simulink model "sm_car_Unreal_Engine_test_transforms_R19b"  (R2021b)
settings: Solver=VariableStepAuto  StartTime=0.0  StopTime=20  RelTol=1e-3  EnableMultiTasking=on
undefined symbols (not defined in the file or in its folder): Newton, Raphson, X, Y, Z
libraries: sm_lib x18, nesl_utility x9, sharedtransformsys x3, sim3dlib x1, sim3dautolib x1, Vehicle_Visualization x1
Description:
  | Copyright 2020-2021 The MathWorks, Inc.
settings Model: Creator=bmirtich  LastModifiedBy=smiller
settings SolverCC: AlgebraicLoopSolver=TrustRegion
settings DataIOCC: LimitDataPoints=on  MaxDataPoints=10000
settings OptimizationCC: LifeSpan=inf
settings DebuggingCC: ParameterPrecisionLossMsg=none  ParameterTunabilityLossMsg=none  AllowSymbolicDim=off  SFUnexpectedBacktrackingDiag=warning  SFNoUnconditionalDefaultTransitionDiag=warning  SFExecutionAtInitializationDiag=none  SFMachineParentedDataDiag=warning  ArithmeticOperatorsInVariantConditions=warning
settings SFSimCC: SimUseLocalCustomCode=off  CustomCodeUndefinedFunction=UseInterfaceOnly
settings RTWCC: RTWUseLocalCustomCode=off
settings CodeAppCC: StateflowObjectComments=on
settings GRTTargetCC: TargetLangStandard=C89/C90 (ANSI)
settings ConfigComp: CovMetricSettings=dw  CovSaveCumulativeToWorkspaceVar=on  CovSaveSingleToWorkspaceVar=on  CovExternalEMLEnable=off  CovSFcnEnable=off
settings SimscapeCC: SimscapeLogType=all  SimscapeLogSimulationStatistics=on  SimscapeLogDataHistory=10000
settings DiagnosticsConfigSet: SimMechanicsConflictingReferenceFrames=none
settings ExplorerConfigSet: InternalSimMechanicsExplorerSettings="<ExplorerConfiguration><canonicalview>default</canonicalview><AnimationSetting><BasePlaybackSpeed>1.0</BasePlaybackSpeed><PlaybackSpeedFactor>2.0</PlaybackSpeedFactor></AnimationSetting><TilePanel><TileInfo><Tiles Columns=\"1\" Count=\"1\" Rows=\"1\"><Column Weight=\"1\"/><Row Weight=\"1\"/><Tile Height=\"1\" Width=\"1\" X=\"0\" Y=\"0\"/></Tiles></TileInfo><SceneInfo><SceneViewer><BGColor><R>1</R><G>1</G><B>1</B></BGColor><Camera><DoPerspective>on</DoPerspective><Position><X>-10</X><Y>0</Y><Z>1</Z></Position><Center><X>-9</X><Y>0</Y><Z>1</Z></Center><Up><X>0</X><Y>0</Y><Z>1</Z></Up><ViewLimDist>1</ViewLimDist><YLim>0.466307658154998583</YLim><XLim>0.637328144918969053</XLim></Camera></SceneViewer></SceneInfo></TilePanel><MechEditorPanel><Cameras><Camera><Id>Camera8</Id><Value><Name>Track Align Rear STL</Name><NativeCamera><PositionTrackingFeature>Vehicle_Geometry.Transform_Camera_Rear.F</PositionTrackingFeature><CenterTrackingFeature>Vehicle_Geometry.Transform_Camera_Rear.F</CenterTrackingFeature><UpVectorTrackingFeature>Vehicle_Geometry.Transform_Camera_Rear.F</UpVectorTrackingFeature><CenterTrackingOrigin>off</CenterTrackingOrigin><CenterTrackingDirection>+X</CenterTrackingDirection><UpVectorTrackingDirection>+Z</UpVectorTrackingDirection></NativeCamera></Value></Camera><Camera><Id>Camera9</Id><Value><Name>Track Rear Fixed View</Name><NativeCamera><PositionTrackingFeature>Ground_Plane.Transform_Camera_Fixed.F</PositionTrackingFeature><CenterTrackingFeature>Ground_Plane.Transform_Camera_Fixed.F</CenterTrackingFeature><UpVectorTrackingFeature>Ground_Plane.Transform_Camera_Fixed.F</UpVectorTrackingFeature><CenterTrackingOrigin>off</CenterTrackingOrigin><CenterTrackingDirection>+X</CenterTrackingDirection><UpVectorTrackingDirection>+Z</UpVectorTrackingDirection></NativeCamera></Value></Camera></Cameras><GfxPanelCameraMap><MapElement CameraMLId=\"Camera9\" GfxPanelIndex=\"0\"/></GfxPanelCameraMap><VideoCreator><PlaybackSpeedRatio>1.0</PlaybackSpeedRatio><FrameRate>30</FrameRate><VideoFormat>Motion JPEG AVI</VideoFormat><FrameSize>auto</FrameSize></VideoCreator></MechEditorPanel></ExplorerConfiguration>"

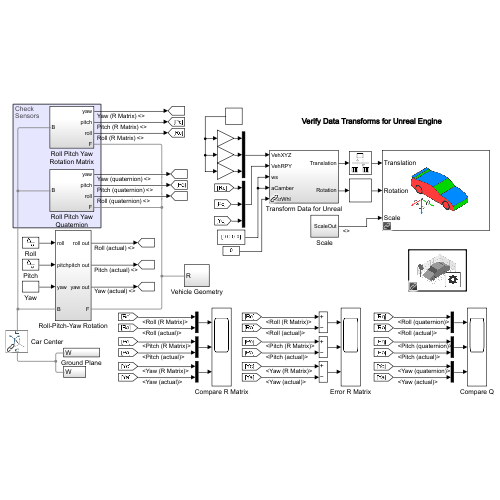
[thumbnail: Simulink's stored preview of the top-level diagram]
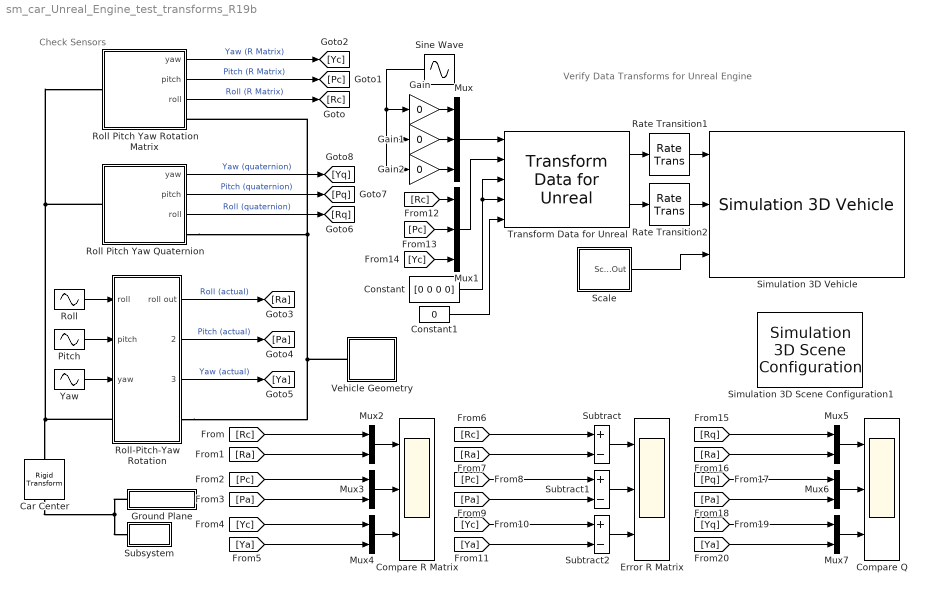
== system sm_car_Unreal_Engine_test_transforms_R19b ==
  note: Check
      | Sensors
  note: Verify Data Transforms for Unreal Engine
  Car Center : sm_lib/Frames and Transforms/Rigid Transform  TranslationMethod=Cartesian  TranslationStandardOffset=0  TranslationLengthUnit=m  TranslationStandardAxis=+Z  TranslationCartesianOffset=[0 0 .85]  TranslationROffset=0  TranslationROffsetUnits=m  TranslationZOffset=0  TranslationZOffsetUnits=m  TranslationThetaOffset=0  TranslationThetaOffsetUnits=deg  RotationMethod=None  RotationAngleUnits=deg  RotationStandardAxis=+Z  RotationAngle=0.0  RotationArbitraryAxis=[0 0 1]  FollAlignAxisA=+X  BaseAlignAxisA=+Y  FollAlignAxisB=+Y  BaseAlignAxisB=+Z  RotationSequenceAxes=FollowerAxes  RotationSequence=XYX  RotationSequenceAngles=[0 0 0]  RotationSequenceAnglesUnits=deg  RotationMatrix=[1 0 0; 0 1 0; 0 0 1]
      settings: SourceProductName=Multibody
  Compare Q : Scope  NumInputPorts=3
  Compare R Matrix : Scope  NumInputPorts=3
  Constant : Constant  Value=[0 0 0 0]
  Constant1 : Constant  Value=0
  Error R Matrix : Scope  NumInputPorts=3
  Gain : Gain  Gain=0
  Gain1 : Gain  Gain=0
  Gain2 : Gain  Gain=0
  Ground Plane : Subsystem
  Mux : Mux  Inputs=3
  Mux1 : Mux  Inputs=3
  Mux{2..7} (6 alike) : Mux  Inputs=2
  Pitch : Sin  Amplitude=80  Frequency=1.329  SampleTime=0
  Rate Transition1 : RateTransition  Deterministic=off  OutPortSampleTime=0.03
  Rate Transition2 : RateTransition  Deterministic=off  OutPortSampleTime=0.03
  Roll : Sin  Amplitude=150  Frequency=.991  SampleTime=0
  Roll Pitch Yaw Quaternion : Subsystem
  Roll Pitch Yaw Rotation Matrix : Subsystem
  Roll-Pitch-Yaw Rotation : Subsystem
  Scale : Subsystem
  Simulation 3D Scene Configuration1 : sim3dlib/Simulation 3D Scene Configuration  Priority=0  ProjectFormat_internal=Default Scenes  ProjectFormat=Default Scenes  SceneDesc=Double lane change  ProjectName=C:\Program Files\MATLAB\R2021b\toolbox\shared\sim3d_projects\automotive_project\UE4\WindowsNoEditor\VehicleSimulation.exe  ScenePath=/Game/Maps/HwStrght  vehTagList={'Scene Origin'}  vehTag=Scene Origin  OpVisEn=off  Ts=.03  EnableWindow=on  EnableWeather=off  SunAltitude=40.0  SunAzimuth=90  clouds=10  wind=1  fog=0  rain=0  sensorTag=MainCamera1  sensorId=1  sensorName=MainCamera1  mountLoc=Origin  offsetFlag=off  tmountOffset=[0, 0, 0]  rmountOffset=[0, 0, 0]  HorizontalResolution=1280  VerticalResolution=720  HorizontalFOV=60  mountPoint=[0 0 0]  mountOrientation=[0 0 0]  aMode=aMode  ID=1
      settings: SourceProductBaseCode=AE,DR,UV,VE
  Simulation 3D Vehicle : sim3dautolib/Simulation 3D Vehicle  Priority=-1  PassVehMesh=Muscle car  PassVehMesh_Internal=Muscle car  MeshPath=/MathWorksSimulation/Vehicles/Muscle/Meshes/SK_MuscleCar.SK_MuscleCar  VehColor=Red  VehColor_Internal=Red  ActorName=SimulinkVehicle1  VehLightsControl=off  HeadlightColor=[ 1, 1, 1 ]  HighBeamIntensity=100000  LowBeamIntensity=60000  HighBeamConeAngle=1.22  LowBeamConeAngle=1.22  LeftHeadlightOrientation=[ 0, 0 ]  RightHeadlightOrientation=[ 0, 0 ]  BrakelightIntensity=500  ReverselightIntensity=500  SignallightIntensity=500  SignallightPeriod=1  SignalPulseWidth=50  Translation=[0 0 1; 0 0 0; 0 0 0; 0 0 0; 0 0 0]  Rotation=[0 0 0; 0 0 0; 0 0 0; 0 0 0; 0 0 0]  Scale=ones( 5, 3 )  SampleTime=.03  ActorType=SimulinkVehicle  ID=1  aMode=2  ActorTag=SimulinkVehicle1
      settings: SourceProductBaseCode=AE,DR,UV,VE
  Sine Wave : Sin  SampleTime=0
  Subsystem : Subsystem
  Subtract : Sum  Inputs=+-
  Subtract1 : Sum  Inputs=+-
  Subtract2 : Sum  Inputs=+-
  Transform Data for Unreal : Vehicle_Visualization/Transform Data for Unreal  SystemSampleTime=-1  VariantActivationTime=update diagram  Latency=0  AutoFrameSizeCalculation=off
  Vehicle Geometry : Subsystem
  Yaw : Sin  Amplitude=130  Frequency=.543  SampleTime=0
  wires:
  Roll Pitch Yaw Rotation Matrix/2(pitch) -> [Pc]  "Pitch (R Matrix)"
  Roll/1 -> Roll-Pitch-Yaw Rotation/1(roll)
  Roll-Pitch-Yaw Rotation/2(pitch out) -> [Pa]  "Pitch (actual)"
  Pitch/1 -> Roll-Pitch-Yaw Rotation/2(pitch)
  Yaw/1 -> Roll-Pitch-Yaw Rotation/3(yaw)
  Roll-Pitch-Yaw Rotation/3(yaw out) -> [Ya]  "Yaw (actual)"
  Roll Pitch Yaw Rotation Matrix/1(yaw) -> [Yc]  "Yaw (R Matrix)"
  Roll-Pitch-Yaw Rotation/1(roll out) -> [Ra]  "Roll (actual)"
  [Rc] -> Mux2/1
  Roll Pitch Yaw Rotation Matrix/3(roll) -> [Rc]  "Roll (R Matrix)"
  [Ra] -> Mux2/2
  [Pc] -> Mux3/1
  [Pa] -> Mux3/2
  [Yc] -> Mux4/1
  [Ya] -> Mux4/2
  [Yc] -> Subtract2/1
  [Pa] -> Subtract1/2
  [Pc] -> Subtract1/1
  [Ya] -> Subtract2/2
  [Rc] -> Subtract/1
  [Ra] -> Subtract/2
  Subtract/1 -> Error R Matrix/1
  Subtract1/1 -> Error R Matrix/2
  Subtract2/1 -> Error R Matrix/3
  Scale/1(ScaleOut) -> Simulation 3D Vehicle/3
  Transform Data for Unreal/2 -> Rate Transition2/1
  Rate Transition1/1 -> Simulation 3D Vehicle/1
  Rate Transition2/1 -> Simulation 3D Vehicle/2
  Transform Data for Unreal/1 -> Rate Transition1/1
  Gain1/1 -> Mux/2
  Gain/1 -> Mux/1
  Sine Wave/1 -> Gain2/1, Gain1/1, Gain/1
  Gain2/1 -> Mux/3
  [Rc] -> Mux1/1
  [Pc] -> Mux1/2
  [Yc] -> Mux1/3
  Mux/1 -> Transform Data for Unreal/1
  Mux1/1 -> Transform Data for Unreal/2
  Constant/1 -> Transform Data for Unreal/4, Transform Data for Unreal/3
  Constant1/1 -> Transform Data for Unreal/5
  Mux4/1 -> Compare R Matrix/3
  Mux2/1 -> Compare R Matrix/1
  Mux3/1 -> Compare R Matrix/2
  Roll Pitch Yaw Quaternion/3(roll) -> [Rq]  "Roll (quaternion)"
  Roll Pitch Yaw Quaternion/1(yaw) -> [Yq]  "Yaw (quaternion)"
  Roll Pitch Yaw Quaternion/2(pitch) -> [Pq]  "Pitch (quaternion)"
  Mux6/1 -> Compare Q/2
  Mux5/1 -> Compare Q/1
  Mux7/1 -> Compare Q/3
  [Ya] -> Mux7/2
  [Yq] -> Mux7/1
  [Pa] -> Mux6/2
  [Pq] -> Mux6/1
  [Ra] -> Mux5/2
  [Rq] -> Mux5/1
  connections:
  Roll-Pitch-Yaw Rotation/RConn1 -- Vehicle Geometry/LConn1 -- Roll Pitch Yaw Rotation Matrix/RConn1 -- Roll Pitch Yaw Quaternion/RConn1
  Roll-Pitch-Yaw Rotation/LConn1 -- Car Center/RConn1 -- Roll Pitch Yaw Quaternion/LConn1 -- Roll Pitch Yaw Rotation Matrix/LConn1
  Car Center/LConn1 -- Ground Plane/LConn1 -- Subsystem/LConn1

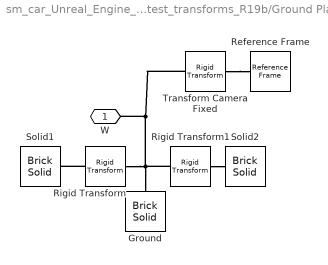
== system sm_car_Unreal_Engine_test_transforms_R19b/Ground Plane ==
  Ground : sm_lib/Body Elements/Brick Solid  GraphicAmbientColor=[0.15 0.15 0.15 1.0]  BasedOnType=Density  BrickDimensions=[100 100 .1]  BrickDimensionUnits=m  CenterOfMass=[0 0 0]  CenterOfMassUnits=m  GraphicDiffuseColor=[0.5 0.5 0.5]  Density=1000  DensityUnits=kg/m^3  DoExposeReferenceFrame=on  GraphicEmissiveColor=[0.0 0.0 0.0 1.0]  ExportEntireGeometry=off  SerializedFrames=<Frames/>  MarkerShape=Sphere  MarkerSize=10  GraphicType=FromGeometry  InertiaType=CalculateFromGeometry  Mass=1  MassUnits=kg  MomentsOfInertia=[1 1 1]  MomentsOfInertiaUnits=kg*m^2  GraphicOpacity=0.5  ProductsOfInertia=[0 0 0]  ProductsOfInertiaUnits=kg*m^2  GraphicShininess=75  GraphicSpecularColor=[0.5 0.5 0.5 1.0]  GraphicVisPropType=SimpleVisualProperties
  Reference Frame : sm_lib/Frames and Transforms/Reference Frame
  Rigid Transform : sm_lib/Frames and Transforms/Rigid Transform  TranslationMethod=StandardAxis  TranslationStandardOffset=1.5  TranslationLengthUnit=m  TranslationStandardAxis=+Y  TranslationCartesianOffset=[0 0 0]  TranslationROffset=0  TranslationROffsetUnits=m  TranslationZOffset=0  TranslationZOffsetUnits=m  TranslationThetaOffset=0  TranslationThetaOffsetUnits=deg  RotationMethod=None  RotationAngleUnits=deg  RotationStandardAxis=+Z  RotationAngle=0.0  RotationArbitraryAxis=[0 0 1]  FollAlignAxisA=+X  BaseAlignAxisA=+Y  FollAlignAxisB=+Y  BaseAlignAxisB=+Z  RotationSequenceAxes=FollowerAxes  RotationSequence=XYX  RotationSequenceAngles=[0 0 0]  RotationSequenceAnglesUnits=deg  RotationMatrix=[1 0 0; 0 1 0; 0 0 1]
  Rigid Transform1 : sm_lib/Frames and Transforms/Rigid Transform  TranslationMethod=StandardAxis  TranslationStandardOffset=1.5  TranslationLengthUnit=m  TranslationStandardAxis=+Y  TranslationCartesianOffset=[0 0 0]  TranslationROffset=0  TranslationROffsetUnits=m  TranslationZOffset=0  TranslationZOffsetUnits=m  TranslationThetaOffset=0  TranslationThetaOffsetUnits=deg  RotationMethod=None  RotationAngleUnits=deg  RotationStandardAxis=+Z  RotationAngle=0.0  RotationArbitraryAxis=[0 0 1]  FollAlignAxisA=+X  BaseAlignAxisA=+Y  FollAlignAxisB=+Y  BaseAlignAxisB=+Z  RotationSequenceAxes=FollowerAxes  RotationSequence=XYX  RotationSequenceAngles=[0 0 0]  RotationSequenceAnglesUnits=deg  RotationMatrix=[1 0 0; 0 1 0; 0 0 1]
  Solid1 : sm_lib/Body Elements/Brick Solid  GraphicAmbientColor=[0.15 0.15 0.15 1.0]  BasedOnType=Density  BrickDimensions=[100 0.11 0.11]  BrickDimensionUnits=m  CenterOfMass=[0 0 0]  CenterOfMassUnits=m  GraphicDiffuseColor=[1.0 1.0 0.2]  Density=1000  DensityUnits=kg/m^3  DoExposeReferenceFrame=on  GraphicEmissiveColor=[0.0 0.0 0.0 1.0]  ExportEntireGeometry=off  SerializedFrames=<Frames/>  MarkerShape=Sphere  MarkerSize=10  GraphicType=FromGeometry  InertiaType=CalculateFromGeometry  Mass=1  MassUnits=kg  MomentsOfInertia=[1 1 1]  MomentsOfInertiaUnits=kg*m^2  GraphicOpacity=1.0  ProductsOfInertia=[0 0 0]  ProductsOfInertiaUnits=kg*m^2  GraphicShininess=75  GraphicSpecularColor=[0.5 0.5 0.5 1.0]  GraphicVisPropType=SimpleVisualProperties
  Solid2 : sm_lib/Body Elements/Brick Solid  GraphicAmbientColor=[0.15 0.15 0.15 1.0]  BasedOnType=Density  BrickDimensions=[100 0.11 0.11]  BrickDimensionUnits=m  CenterOfMass=[0 0 0]  CenterOfMassUnits=m  GraphicDiffuseColor=[1.0 1.0 1.0]  Density=1000  DensityUnits=kg/m^3  DoExposeReferenceFrame=on  GraphicEmissiveColor=[0.0 0.0 0.0 1.0]  ExportEntireGeometry=off  SerializedFrames=<Frames/>  MarkerShape=Sphere  MarkerSize=10  GraphicType=FromGeometry  InertiaType=CalculateFromGeometry  Mass=1  MassUnits=kg  MomentsOfInertia=[1 1 1]  MomentsOfInertiaUnits=kg*m^2  GraphicOpacity=1.0  ProductsOfInertia=[0 0 0]  ProductsOfInertiaUnits=kg*m^2  GraphicShininess=75  GraphicSpecularColor=[0.5 0.5 0.5 1.0]  GraphicVisPropType=SimpleVisualProperties
  Transform Camera Fixed : sm_lib/Frames and Transforms/Rigid Transform  TranslationMethod=Cartesian  TranslationStandardOffset=0  TranslationLengthUnit=m  TranslationStandardAxis=+Z  TranslationCartesianOffset=[-10 0 1]  TranslationROffset=0  TranslationROffsetUnits=m  TranslationZOffset=0  TranslationZOffsetUnits=m  TranslationThetaOffset=0  TranslationThetaOffsetUnits=deg  RotationMethod=None  RotationAngleUnits=deg  RotationStandardAxis=+Z  RotationAngle=0.0  RotationArbitraryAxis=[0 0 1]  FollAlignAxisA=+X  BaseAlignAxisA=+Y  FollAlignAxisB=+Y  BaseAlignAxisB=+Z  RotationSequenceAxes=FollowerAxes  RotationSequence=XYX  RotationSequenceAngles=[0 0 0]  RotationSequenceAnglesUnits=deg  RotationMatrix=[1 0 0; 0 1 0; 0 0 1]
  W : PMIOPort  Side=Left
  connections:
  Rigid Transform/RConn1 -- Solid1/RConn1
  Rigid Transform1/LConn1 -- Solid2/RConn1
  Rigid Transform/LConn1 -- Transform Camera Fixed/LConn1 -- W/RConn1 -- Rigid Transform1/RConn1 -- Ground/RConn1
  Transform Camera Fixed/RConn1 -- Reference Frame/RConn1

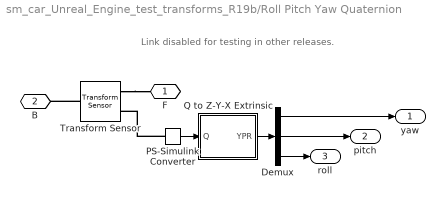
== system sm_car_Unreal_Engine_test_transforms_R19b/Roll Pitch Yaw Quaternion ==
  note: Link disabled for testing in other releases.
  Demux : Demux  Outputs=3
  PS-Simulink Converter : nesl_utility/PS-Simulink Converter  PhysicalDomain=network_engine_domain  SubClassName=ps_output  LeftPortType=input  RightPortType=output  PseudoPeriodic=off  Frequencies=[]  Unit=1  AffineConversion=off
      settings: SourceProductBaseCode=PW,SS
  Q to Z-Y-X Extrinsic : Subsystem  AncestorBlock=sm_car_lib/Utilities/Q to Z-Y-X Extrinsic
  Transform Sensor : sm_lib/Frames and Transforms/Transform Sensor  MeasurementFrame=Base  SenseAngle=off  SenseAxis=off  SenseAngle1=off  SenseAngle2=off  SenseAngle3=off  SenseQ=on  SenseR=off  SenseOmegaX=off  SenseOmegaY=off  SenseOmegaZ=off  SenseOmega1=off  SenseOmega2=off  SenseOmega3=off  SenseQDot=off  SenseRDot=off  SenseAlphaX=off  SenseAlphaY=off  SenseAlphaZ=off  SenseAlpha1=off  SenseAlpha2=off  SenseAlpha3=off  SenseQDDot=off  SenseRDDot=off  SenseX=off  SenseY=off  SenseZ=off  SenseRad=off  SenseAzim=off  SenseDist=off  SenseInc=off  SenseXDot=off  SenseYDot=off  SenseZDot=off  SenseRadDot=off  SenseAzimDot=off  SenseDistDot=off  SenseIncDot=off  SenseXDDot=off  SenseYDDot=off  SenseZDDot=off  SenseRadDDot=off  SenseAzimDDot=off  SenseDistDDot=off  SenseIncDDot=off
  F : PMIOPort  Side=Right
  B : PMIOPort  Port=2  Side=Left
  yaw : Outport  VectorParamsAs1DForOutWhenUnconnected=off
  pitch : Outport  Port=2  VectorParamsAs1DForOutWhenUnconnected=off
  roll : Outport  Port=3  VectorParamsAs1DForOutWhenUnconnected=off
  wires:
  Demux/2 -> pitch/1
  Demux/3 -> roll/1
  Demux/1 -> yaw/1
  PS-Simulink Converter/1 -> Q to Z-Y-X Extrinsic/1(Q)
  Q to Z-Y-X Extrinsic/1(YPR) -> Demux/1
  connections:
  Transform Sensor/RConn1 -- F/RConn1
  Transform Sensor/LConn1 -- B/RConn1
  PS-Simulink Converter/LConn1 -- Transform Sensor/RConn2

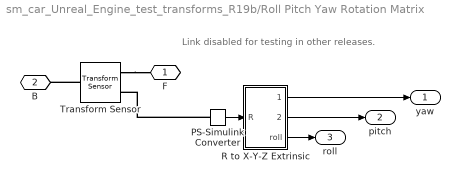
== system sm_car_Unreal_Engine_test_transforms_R19b/Roll Pitch Yaw Rotation Matrix ==
  note: Link disabled for testing in other releases.
  PS-Simulink Converter : nesl_utility/PS-Simulink Converter  PhysicalDomain=network_engine_domain  SubClassName=ps_output  LeftPortType=input  RightPortType=output  PseudoPeriodic=off  Frequencies=[]  Unit=1  AffineConversion=off
      settings: SourceProductBaseCode=PW,SS
  R to X-Y-Z Extrinsic : Subsystem  AncestorBlock=sm_car_lib/Body/Body to World/R to X-Y-Z Extrinsic
  Transform Sensor : sm_lib/Frames and Transforms/Transform Sensor  MeasurementFrame=Base  SenseAngle=off  SenseAxis=off  SenseAngle1=off  SenseAngle2=off  SenseAngle3=off  SenseQ=off  SenseR=on  SenseOmegaX=off  SenseOmegaY=off  SenseOmegaZ=off  SenseOmega1=off  SenseOmega2=off  SenseOmega3=off  SenseQDot=off  SenseRDot=off  SenseAlphaX=off  SenseAlphaY=off  SenseAlphaZ=off  SenseAlpha1=off  SenseAlpha2=off  SenseAlpha3=off  SenseQDDot=off  SenseRDDot=off  SenseX=off  SenseY=off  SenseZ=off  SenseRad=off  SenseAzim=off  SenseDist=off  SenseInc=off  SenseXDot=off  SenseYDot=off  SenseZDot=off  SenseRadDot=off  SenseAzimDot=off  SenseDistDot=off  SenseIncDot=off  SenseXDDot=off  SenseYDDot=off  SenseZDDot=off  SenseRadDDot=off  SenseAzimDDot=off  SenseDistDDot=off  SenseIncDDot=off
  F : PMIOPort  Side=Right
  B : PMIOPort  Port=2  Side=Left
  yaw : Outport  VectorParamsAs1DForOutWhenUnconnected=off
  pitch : Outport  Port=2  VectorParamsAs1DForOutWhenUnconnected=off
  roll : Outport  Port=3  VectorParamsAs1DForOutWhenUnconnected=off
  wires:
  PS-Simulink Converter/1 -> R to X-Y-Z Extrinsic/1(R)
  R to X-Y-Z Extrinsic/1(yaw) -> yaw/1
  R to X-Y-Z Extrinsic/3(roll) -> roll/1
  R to X-Y-Z Extrinsic/2(pitch) -> pitch/1
  connections:
  PS-Simulink Converter/LConn1 -- Transform Sensor/RConn2
  Transform Sensor/LConn1 -- B/RConn1
  Transform Sensor/RConn1 -- F/RConn1

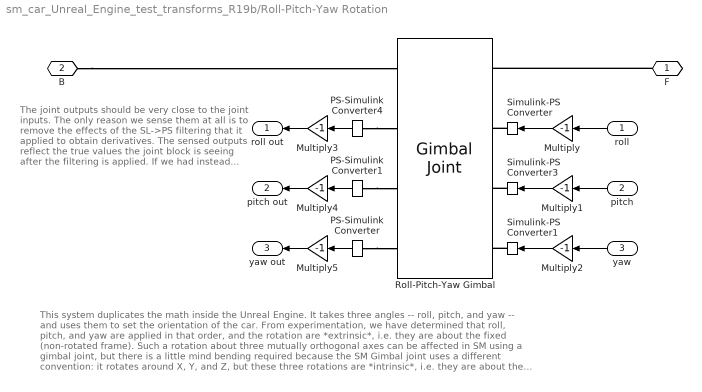
== system sm_car_Unreal_Engine_test_transforms_R19b/Roll-Pitch-Yaw Rotation ==
  note: The joint outputs should be very close to the joint inputs. The only reason we sense them at all is to remove the effects of the SL->PS filtering that it applied to obtain derivatives. The sensed outputs reflect the true values the joint block is seeing after the filtering is applied. If we had instead compared the computed roll/pitch/yaw to the roll/pitch/yaw values being fed into this block, the errors would be slightly greater because of the filtering.
  note: This system duplicates the math inside the Unreal Engine. It takes three angles -- roll, pitch, and yaw -- and uses them to set the orientation of the car. From experimentation, we have determined that roll, pitch, and yaw are applied in that order, and the rotation are *extrinsic*, i.e. they are about the fixed (non-rotated frame).
      |
      | Such a rotation about three mutually orthogonal axes can be affected in SM using a gimbal joint, but there is a little mind bending required because the SM Gimbal joint uses a different convention: it rotates around X, Y, and Z, but these three rotations are *intrinsic*, i.e. they are about the rotated axes. Nonetheless, the extrinsic rotations can be implemented with the intrinsic gimbal joint by: (1) reverseing the direction of the joint (note the reversed B/F connections above), and (2) negating the angles provided to the joint. When this is done, it can be shown that the gimbal performs an extrinsic X, Y, Z rotation.
      |
      | See https://en.wikipedia.org/wiki/Euler_angles for more information on Euler angles.
  roll : Inport
  pitch : Inport  Port=2
  yaw : Inport  Port=3
  Multiply{,1..5} (6 alike) : Gain  Gain=-1
  PS-Simulink Converter : nesl_utility/PS-Simulink Converter  PhysicalDomain=network_engine_domain  SubClassName=ps_output  LeftPortType=input  RightPortType=output  PseudoPeriodic=off  Frequencies=[]  Unit=rad  AffineConversion=off
      settings: SourceProductName=Utilities
  PS-Simulink Converter1 : nesl_utility/PS-Simulink Converter  PhysicalDomain=network_engine_domain  SubClassName=ps_output  LeftPortType=input  RightPortType=output  PseudoPeriodic=off  Frequencies=[]  Unit=rad  AffineConversion=off
      settings: SourceProductName=Utilities
  PS-Simulink Converter4 : nesl_utility/PS-Simulink Converter  PhysicalDomain=network_engine_domain  SubClassName=ps_output  LeftPortType=input  RightPortType=output  PseudoPeriodic=off  Frequencies=[]  Unit=rad  AffineConversion=off
      settings: SourceProductName=Utilities
  Roll-Pitch-Yaw Gimbal : sm_lib/Joints/Gimbal Joint  JointMode=Normal  SenseConstraintForce=off  SenseConstraintForceX=off  SenseConstraintForceY=off  SenseConstraintForceZ=off  SenseConstraintTorque=off  SenseConstraintTorqueX=off  SenseConstraintTorqueY=off  SenseConstraintTorqueZ=off  SenseTotalForce=off  SenseTotalForceX=off  SenseTotalForceY=off  SenseTotalForceZ=off  SenseTotalTorque=off  SenseTotalTorqueX=off  SenseTotalTorqueY=off  SenseTotalTorqueZ=off  CompositeWrenchDir=FollowerOnBase  CompositeWrenchFrame=BaseFrame  RxEquilibriumPosition=0  RxEquilibriumPositionUnits=deg  RxSpringStiffness=0  RxSpringStiffnessUnits=N*m/deg  RxDampingCoefficient=0  RxDampingCoefficientUnits=N*m/(deg/s)  RxTorqueActuationMode=ComputedTorque  RxMotionActuationMode=InputMotion  RxSensePosition=on  RxSenseVelocity=off  RxSenseAcceleration=off  RxSenseTorqueForce=off  RxSenseLowerLimitTorqueForce=off  RxSenseUpperLimitTorqueForce=off  RxLowerLimitSpecify=off  RxLowerLimitBound=-90  RxLowerLimitBoundUnits=deg  RxLowerLimitStiffness=1e4  RxLowerLimitStiffnessUnits=N*m/deg  RxLowerLimitDamping=10  RxLowerLimitDampingUnits=N*m/(deg/s)  RxLowerLimitTransitionRegionWidth=0.1  RxLowerLimitTransitionRegionWidthUnits=deg  RxUpperLimitSpecify=off  RxUpperLimitBound=90  RxUpperLimitBoundUnits=deg  RxUpperLimitStiffness=1e4  RxUpperLimitStiffnessUnits=N*m/deg  RxUpperLimitDamping=10  RxUpperLimitDampingUnits=N*m/(deg/s)  RxUpperLimitTransitionRegionWidth=0.1  RxUpperLimitTransitionRegionWidthUnits=deg  RxPositionTargetSpecify=off  RxPositionTargetPriority=High  RxPositionTargetValue=0  RxPositionTargetValueUnits=deg  RxVelocityTargetSpecify=off  RxVelocityTargetPriority=High  RxVelocityTargetValue=0  RxVelocityTargetValueUnits=deg/s  RyEquilibriumPosition=0  RyEquilibriumPositionUnits=deg  RySpringStiffness=0  RySpringStiffnessUnits=N*m/deg  RyDampingCoefficient=0  RyDampingCoefficientUnits=N*m/(deg/s)  RyTorqueActuationMode=ComputedTorque  RyMotionActuationMode=InputMotion  RySensePosition=on  RySenseVelocity=off  RySenseAcceleration=off  RySenseTorqueForce=off  RySenseLowerLimitTorqueForce=off  RySenseUpperLimitTorqueForce=off  RyLowerLimitSpecify=off  RyLowerLimitBound=-90  RyLowerLimitBoundUnits=deg  RyLowerLimitStiffness=1e4  RyLowerLimitStiffnessUnits=N*m/deg  RyLowerLimitDamping=10  RyLowerLimitDampingUnits=N*m/(deg/s)  RyLowerLimitTransitionRegionWidth=0.1  RyLowerLimitTransitionRegionWidthUnits=deg  RyUpperLimitSpecify=off  RyUpperLimitBound=90  RyUpperLimitBoundUnits=deg  RyUpperLimitStiffness=1e4  RyUpperLimitStiffnessUnits=N*m/deg  RyUpperLimitDamping=10  RyUpperLimitDampingUnits=N*m/(deg/s)  RyUpperLimitTransitionRegionWidth=0.1  RyUpperLimitTransitionRegionWidthUnits=deg  RyPositionTargetSpecify=off  RyPositionTargetPriority=High  RyPositionTargetValue=0  RyPositionTargetValueUnits=deg  RyVelocityTargetSpecify=off  RyVelocityTargetPriority=High  RyVelocityTargetValue=0  RyVelocityTargetValueUnits=deg/s  RzEquilibriumPosition=0  RzEquilibriumPositionUnits=deg  RzSpringStiffness=0  RzSpringStiffnessUnits=N*m/deg  RzDampingCoefficient=0  RzDampingCoefficientUnits=N*m/(deg/s)  RzTorqueActuationMode=ComputedTorque  RzMotionActuationMode=InputMotion  RzSensePosition=on  RzSenseVelocity=off  RzSenseAcceleration=off  RzSenseTorqueForce=off  RzSenseLowerLimitTorqueForce=off  RzSenseUpperLimitTorqueForce=off  RzLowerLimitSpecify=off  RzLowerLimitBound=-90  RzLowerLimitBoundUnits=deg  RzLowerLimitStiffness=1e4  RzLowerLimitStiffnessUnits=N*m/deg  RzLowerLimitDamping=10  RzLowerLimitDampingUnits=N*m/(deg/s)  RzLowerLimitTransitionRegionWidth=0.1  RzLowerLimitTransitionRegionWidthUnits=deg  RzUpperLimitSpecify=off  RzUpperLimitBound=90  RzUpperLimitBoundUnits=deg  RzUpperLimitStiffness=1e4  RzUpperLimitStiffnessUnits=N*m/deg  RzUpperLimitDamping=10  RzUpperLimitDampingUnits=N*m/(deg/s)  RzUpperLimitTransitionRegionWidth=0.1  RzUpperLimitTransitionRegionWidthUnits=deg  RzPositionTargetSpecify=off  RzPositionTargetPriority=High  RzPositionTargetValue=0  RzPositionTargetValueUnits=deg  RzVelocityTargetSpecify=off  RzVelocityTargetPriority=High  RzVelocityTargetValue=0  RzVelocityTargetValueUnits=deg/s
      settings: SourceProductName=Multibody
  Simulink-PS Converter : nesl_utility/Simulink-PS Converter  PhysicalDomain=network_engine_domain  SubClassName=ps_input  LeftPortType=input  RightPortType=output  PseudoPeriodic=off  Frequencies=[]  NoiseDistribution=none  NoiseParameters=[]  Unit=deg  AffineConversion=off  FilteringAndDerivatives=filter  SimscapeFilterOrder=2  InputFilterTimeConstant=1e-2  UdotUserProvided=0
      settings: SourceProductName=Utilities
  Simulink-PS Converter1 : nesl_utility/Simulink-PS Converter  PhysicalDomain=network_engine_domain  SubClassName=ps_input  LeftPortType=input  RightPortType=output  PseudoPeriodic=off  Frequencies=[]  NoiseDistribution=none  NoiseParameters=[]  Unit=deg  AffineConversion=off  FilteringAndDerivatives=filter  SimscapeFilterOrder=2  InputFilterTimeConstant=1e-2  UdotUserProvided=0
      settings: SourceProductName=Utilities
  Simulink-PS Converter3 : nesl_utility/Simulink-PS Converter  PhysicalDomain=network_engine_domain  SubClassName=ps_input  LeftPortType=input  RightPortType=output  PseudoPeriodic=off  Frequencies=[]  NoiseDistribution=none  NoiseParameters=[]  Unit=deg  AffineConversion=off  FilteringAndDerivatives=filter  SimscapeFilterOrder=2  InputFilterTimeConstant=1e-2  UdotUserProvided=0
      settings: SourceProductName=Utilities
  F : PMIOPort  Side=Right
  B : PMIOPort  Port=2  Side=Left
  roll out : Outport
  pitch out : Outport  Port=2
  yaw out : Outport  Port=3
  wires:
  Multiply/1 -> Simulink-PS Converter/1
  roll/1 -> Multiply/1
  PS-Simulink Converter4/1 -> Multiply3/1
  PS-Simulink Converter/1 -> Multiply5/1
  Multiply1/1 -> Simulink-PS Converter3/1
  pitch/1 -> Multiply1/1
  PS-Simulink Converter1/1 -> Multiply4/1
  Multiply2/1 -> Simulink-PS Converter1/1
  yaw/1 -> Multiply2/1
  Multiply3/1 -> roll out/1
  Multiply4/1 -> pitch out/1
  Multiply5/1 -> yaw out/1
  connections:
  F/RConn1 -- Roll-Pitch-Yaw Gimbal/LConn1
  B/RConn1 -- Roll-Pitch-Yaw Gimbal/RConn1
  Simulink-PS Converter/RConn1 -- Roll-Pitch-Yaw Gimbal/LConn2
  Simulink-PS Converter3/RConn1 -- Roll-Pitch-Yaw Gimbal/LConn3
  PS-Simulink Converter4/LConn1 -- Roll-Pitch-Yaw Gimbal/RConn2
  PS-Simulink Converter/LConn1 -- Roll-Pitch-Yaw Gimbal/RConn4
  PS-Simulink Converter1/LConn1 -- Roll-Pitch-Yaw Gimbal/RConn3
  Simulink-PS Converter1/RConn1 -- Roll-Pitch-Yaw Gimbal/LConn4

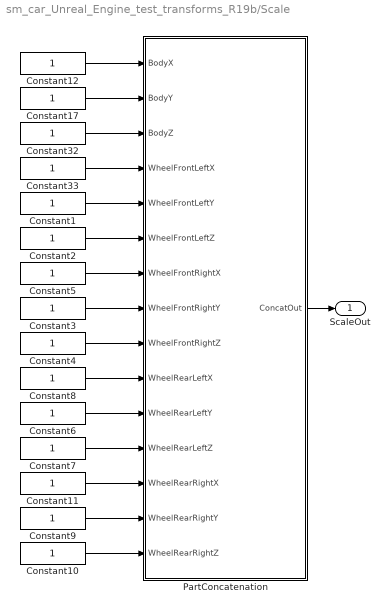
== system sm_car_Unreal_Engine_test_transforms_R19b/Scale ==
  Constant{1..12,17,32..33} (15 alike) : Constant  OutDataTypeStr=single
  PartConcatenation : Subsystem
  ScaleOut : Outport  VectorParamsAs1DForOutWhenUnconnected=off
  wires:
  Constant10/1 -> PartConcatenation/15(WheelRearRightZ)
  Constant9/1 -> PartConcatenation/14(WheelRearRightY)
  Constant11/1 -> PartConcatenation/13(WheelRearRightX)
  Constant7/1 -> PartConcatenation/12(WheelRearLeftZ)
  Constant6/1 -> PartConcatenation/11(WheelRearLeftY)
  Constant8/1 -> PartConcatenation/10(WheelRearLeftX)
  Constant4/1 -> PartConcatenation/9(WheelFrontRightZ)
  Constant3/1 -> PartConcatenation/8(WheelFrontRightY)
  Constant5/1 -> PartConcatenation/7(WheelFrontRightX)
  Constant2/1 -> PartConcatenation/6(WheelFrontLeftZ)
  Constant1/1 -> PartConcatenation/5(WheelFrontLeftY)
  Constant33/1 -> PartConcatenation/4(WheelFrontLeftX)
  Constant32/1 -> PartConcatenation/3(BodyZ)
  Constant17/1 -> PartConcatenation/2(BodyY)
  Constant12/1 -> PartConcatenation/1(BodyX)
  PartConcatenation/1(ConcatOut) -> ScaleOut/1

== system sm_car_Unreal_Engine_test_transforms_R19b/Subsystem ==
  Mechanism Configuration : sm_lib/Utilities/Mechanism Configuration  UniformGravity=Constant  GravityVector=[0 0 -9.80665]  GravityUnits=m/s^2  LinearizationDelta=0.001  JointModeTransitionNonlinearIterations=2
      settings: SourceProductName=Multibody
  Solver Configuration : nesl_utility/Solver Configuration  PhysicalDomain=network_engine_domain  SubClassName=solver  LeftPortType=input  RightPortType=generic  Tones=[]  Harmonics=[]  SimulateNoise=off  Profile=off  UseLocalSampling=off  EnableSwitchedLinearOptims=on  FrequencyDomain=off  UseCCode=off  RelTol=0.001  AbsTol=1e-06  MinStep=1e-09  ToWorkspace=off  RevertToSquareIcSolve=off  NumHomotopyIterations=100  PhasorMode=off  PhasorModeNumHarmonics=1  DoDC=off  ResidualTolerance=1e-09  UseLocalSolver=off  LocalSolverChoice=NE_BACKWARD_EULER_ADVANCER  LocalSolverSampleTime=0.001  DoFixedCost=off  MaxNonlinIter=3  MaxModeIter=2  ComputeImpulses=off  ImpulseIterations=2  LinearAlgebra=Sparse  EquationFormulation=NE_TIME_EF  DelaysMemoryBudget=1024  AutomaticFiltering=on  FilteringTimeConstant=0.001  PartitionStorageMethod=AS_NEEDED  PartitionMemoryBudget=1024  PartitionMethod=FAST
      settings: SourceProductName=Utilities
  World Frame : sm_lib/Frames and Transforms/World Frame
      settings: SourceProductName=Multibody
  W : PMIOPort  Side=Left
  connections:
  Mechanism Configuration/RConn1 -- W/RConn1 -- Solver Configuration/RConn1 -- World Frame/RConn1

== system sm_car_Unreal_Engine_test_transforms_R19b/Vehicle Geometry ==
  Camera Frame Align Rear : sm_lib/Frames and Transforms/Reference Frame
  Transform Body : sm_lib/Frames and Transforms/Rigid Transform  TranslationMethod=Cartesian  TranslationStandardOffset=0  TranslationLengthUnit=m  TranslationStandardAxis=+Z  TranslationCartesianOffset=[0 -0.5 -2.1]  TranslationROffset=0  TranslationROffsetUnits=m  TranslationZOffset=0  TranslationZOffsetUnits=m  TranslationThetaOffset=0  TranslationThetaOffsetUnits=deg  RotationMethod=None  RotationAngleUnits=deg  RotationStandardAxis=+Z  RotationAngle=0.0  RotationArbitraryAxis=[0 0 1]  FollAlignAxisA=+X  BaseAlignAxisA=+Y  FollAlignAxisB=+Y  BaseAlignAxisB=+Z  RotationSequenceAxes=FollowerAxes  RotationSequence=XYX  RotationSequenceAngles=[0 0 0]  RotationSequenceAnglesUnits=deg  RotationMatrix=[1 0 0; 0 1 0; 0 0 1]
  Transform Body Ref : sm_lib/Frames and Transforms/Rigid Transform  TranslationMethod=Cartesian  TranslationStandardOffset=0  TranslationLengthUnit=m  TranslationStandardAxis=+Z  TranslationCartesianOffset=[0.9 1 -0.7]  TranslationROffset=0  TranslationROffsetUnits=m  TranslationZOffset=0  TranslationZOffsetUnits=m  TranslationThetaOffset=0  TranslationThetaOffsetUnits=deg  RotationMethod=RotationSequence  RotationAngleUnits=deg  RotationStandardAxis=+Z  RotationAngle=0.0  RotationArbitraryAxis=[0 0 1]  FollAlignAxisA=+X  BaseAlignAxisA=+Y  FollAlignAxisB=+Y  BaseAlignAxisB=+Z  RotationSequenceAxes=FollowerAxes  RotationSequence=ZXY  RotationSequenceAngles=[-90 90 0]  RotationSequenceAnglesUnits=deg  RotationMatrix=[1 0 0; 0 1 0; 0 0 1]
  Transform Camera Rear : sm_lib/Frames and Transforms/Rigid Transform  TranslationMethod=Cartesian  TranslationStandardOffset=0  TranslationLengthUnit=m  TranslationStandardAxis=+Z  TranslationCartesianOffset=[1 1 10]  TranslationROffset=0  TranslationROffsetUnits=m  TranslationZOffset=0  TranslationZOffsetUnits=m  TranslationThetaOffset=0  TranslationThetaOffsetUnits=deg  RotationMethod=RotationSequence  RotationAngleUnits=deg  RotationStandardAxis=+Z  RotationAngle=0.0  RotationArbitraryAxis=[0 0 1]  FollAlignAxisA=+X  BaseAlignAxisA=+Y  FollAlignAxisB=+Y  BaseAlignAxisB=+Z  RotationSequenceAxes=FollowerAxes  RotationSequence=YXZ  RotationSequenceAngles=[90 -90 0]  RotationSequenceAnglesUnits=deg  RotationMatrix=[1 0 0; 0 1 0; 0 0 1]
  Vehicle Body : sm_lib/Body Elements/File Solid  ExtGeomFileName=sm_vehicle_slalom_vehicle_body.STL  UnitType=Custom  ExtGeomFileUnits=mm  StepReaderType=HEX  ExportConvexHullGeometry=off  InertiaType=Custom  Mass=1  MassUnits=kg  CenterOfMass=[0 0 0]  CenterOfMassUnits=m  MomentsOfInertia=[1 1 1]  MomentsOfInertiaUnits=kg*m^2  ProductsOfInertia=[0 0 0]  ProductsOfInertiaUnits=kg*m^2  BasedOnType=Density  Density=1000  DensityUnits=kg/m^3  DoExposeReferenceFrame=on  SerializedFrames=<Frames/>  GraphicType=FromGeometry  MarkerShape=Sphere  MarkerSize=10  GraphicVisPropType=SimpleVisualProperties  GraphicDiffuseColor=[0.2 0.6 1.0]  GraphicSpecularColor=[0.5 0.5 0.5 1.0]  GraphicAmbientColor=[0.15 0.15 0.15 1.0]  GraphicEmissiveColor=[0.0 0.0 0.0 1.0]  GraphicShininess=75  GraphicOpacity=1.0
  R : PMIOPort  Side=Left
  connections:
  Transform Camera Rear/LConn1 -- Transform Body/LConn1 -- Transform Body Ref/RConn1
  Camera Frame Align Rear/RConn1 -- Transform Camera Rear/RConn1
  Transform Body Ref/LConn1 -- R/RConn1
  Vehicle Body/RConn1 -- Transform Body/RConn1

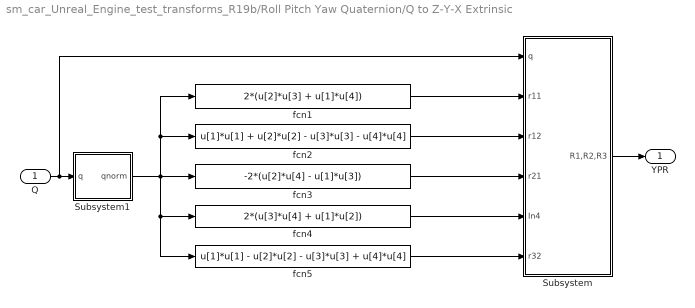
== system sm_car_Unreal_Engine_test_transforms_R19b/Roll Pitch Yaw Quaternion/Q to Z-Y-X Extrinsic ==
  Q : Inport
  Subsystem : Subsystem
  Subsystem1 : Subsystem
  fcn1 : Fcn  Expr=2*(u[2]*u[3] + u[1]*u[4])
  fcn2 : Fcn  Expr=u[1]*u[1] + u[2]*u[2] - u[3]*u[3] - u[4]*u[4]
  fcn3 : Fcn  Expr=-2*(u[2]*u[4] - u[1]*u[3])
  fcn4 : Fcn  Expr=2*(u[3]*u[4] + u[1]*u[2])
  fcn5 : Fcn  Expr=u[1]*u[1] - u[2]*u[2] - u[3]*u[3] + u[4]*u[4]
  YPR : Outport  VectorParamsAs1DForOutWhenUnconnected=off
  wires:
  fcn2/1 -> Subsystem/3(r12)
  fcn4/1 -> Subsystem/5(In4)
  Subsystem1/1(qnorm) -> fcn1/1, fcn2/1, fcn5/1, fcn4/1, fcn3/1
  fcn1/1 -> Subsystem/2(r11)
  fcn3/1 -> Subsystem/4(r21)
  fcn5/1 -> Subsystem/6(r32)
  Q/1 -> Subsystem1/1(q), Subsystem/1(q)
  Subsystem/1(R1,R2,R3) -> YPR/1

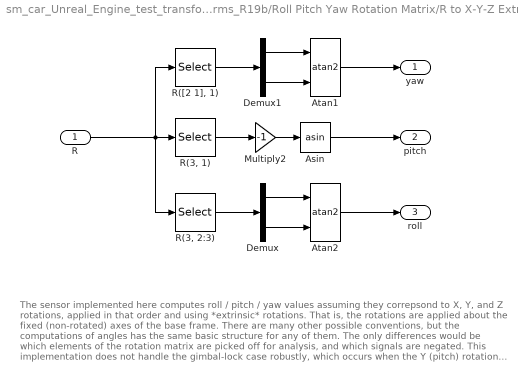
== system sm_car_Unreal_Engine_test_transforms_R19b/Roll Pitch Yaw Rotation Matrix/R to X-Y-Z Extrinsic ==
  note: The sensor implemented here computes roll / pitch / yaw values assuming they correpsond to X, Y, and Z rotations, applied in that order and using  *extrinsic* rotations.  That is, the rotations are applied about the fixed (non-rotated) axes of the base frame.   There are many other possible conventions, but the computations of angles has the same basic structure for any of them.  The only differences would be which elements of the rotation matrix are picked off for analysis, and which signals are negated.
      |
      | This implementation does not handle the gimbal-lock case robustly, which occurs when the Y (pitch) rotation is +/-90 degrees.  Handling this case requires a more complex computation,
      | but it can be done with a few more trig blocks and selectors.
  R : Inport
  Asin : Trigonometry  Operator=asin
  Atan1 : Trigonometry  Operator=atan2
  Atan2 : Trigonometry  Operator=atan2
  Demux : Demux  Outputs=2
  Demux1 : Demux  Outputs=2
  Multiply2 : Gain  Gain=-1
  "R(3, 1)" : Selector  NumberOfDimensions=2  InputPortWidth=3  IndexOptions=Index vector (dialog),Index vector (dialog)  Indices=3,1  OutputSizes=1,1
  "R(3, 2:3)" : Selector  NumberOfDimensions=2  InputPortWidth=3  IndexOptions=Index vector (dialog),Index vector (dialog)  Indices=3,[2 3]  OutputSizes=1,1
  "R([2 1], 1)" : Selector  NumberOfDimensions=2  InputPortWidth=3  IndexOptions=Index vector (dialog),Index vector (dialog)  Indices=[2 1],1  OutputSizes=1,1
  yaw : Outport  VectorParamsAs1DForOutWhenUnconnected=off
  pitch : Outport  Port=2  VectorParamsAs1DForOutWhenUnconnected=off
  roll : Outport  Port=3  VectorParamsAs1DForOutWhenUnconnected=off
  wires:
  Demux/1 -> Atan2/1
  Demux1/2 -> Atan1/2
  Demux/2 -> Atan2/2
  Atan2/1 -> roll/1
  "R(3, 1)"/1 -> Multiply2/1
  Asin/1 -> pitch/1
  R/1 -> "R(3, 1)"/1, "R(3, 2:3)"/1, "R([2 1], 1)"/1
  Demux1/1 -> Atan1/1
  "R([2 1], 1)"/1 -> Demux1/1
  Multiply2/1 -> Asin/1
  "R(3, 2:3)"/1 -> Demux/1
  Atan1/1 -> yaw/1

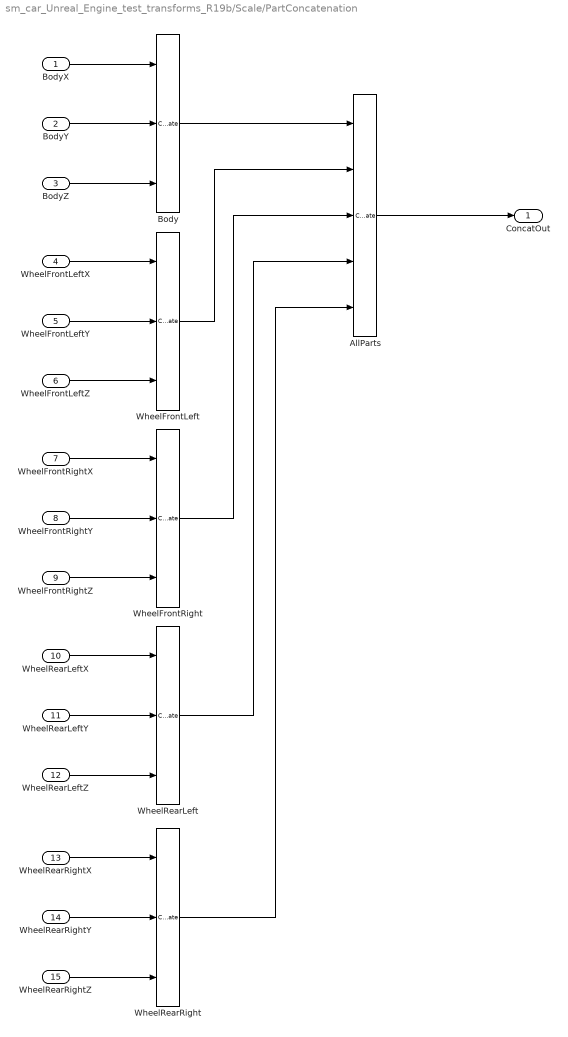
== system sm_car_Unreal_Engine_test_transforms_R19b/Scale/PartConcatenation ==
  BodyX : Inport
  BodyY : Inport  Port=2
  BodyZ : Inport  Port=3
  WheelFrontLeftX : Inport  Port=4
  WheelFrontLeftY : Inport  Port=5
  WheelFrontLeftZ : Inport  Port=6
  WheelFrontRightX : Inport  Port=7
  WheelFrontRightY : Inport  Port=8
  WheelFrontRightZ : Inport  Port=9
  WheelRearLeftX : Inport  Port=10
  WheelRearLeftY : Inport  Port=11
  WheelRearLeftZ : Inport  Port=12
  WheelRearRightX : Inport  Port=13
  WheelRearRightY : Inport  Port=14
  WheelRearRightZ : Inport  Port=15
  AllParts : Concatenate  NumInputs=5  Mode=Multidimensional array
  Body : Concatenate  NumInputs=3  Mode=Multidimensional array  ConcatenateDimension=2
  WheelFrontLeft : Concatenate  NumInputs=3  Mode=Multidimensional array  ConcatenateDimension=2
  WheelFrontRight : Concatenate  NumInputs=3  Mode=Multidimensional array  ConcatenateDimension=2
  WheelRearLeft : Concatenate  NumInputs=3  Mode=Multidimensional array  ConcatenateDimension=2
  WheelRearRight : Concatenate  NumInputs=3  Mode=Multidimensional array  ConcatenateDimension=2
  ConcatOut : Outport  VectorParamsAs1DForOutWhenUnconnected=off
  wires:
  BodyX/1 -> Body/1
  BodyZ/1 -> Body/3
  WheelFrontLeftX/1 -> WheelFrontLeft/1
  WheelFrontLeftZ/1 -> WheelFrontLeft/3
  WheelFrontLeftY/1 -> WheelFrontLeft/2
  BodyY/1 -> Body/2
  WheelFrontLeft/1 -> AllParts/2
  WheelRearRightX/1 -> WheelRearRight/1
  Body/1 -> AllParts/1
  WheelRearLeft/1 -> AllParts/4
  WheelFrontRight/1 -> AllParts/3
  WheelRearRightZ/1 -> WheelRearRight/3
  WheelFrontRightY/1 -> WheelFrontRight/2
  WheelFrontRightX/1 -> WheelFrontRight/1
  WheelRearRightY/1 -> WheelRearRight/2
  WheelRearLeftZ/1 -> WheelRearLeft/3
  AllParts/1 -> ConcatOut/1
  WheelRearLeftY/1 -> WheelRearLeft/2
  WheelRearRight/1 -> AllParts/5
  WheelRearLeftX/1 -> WheelRearLeft/1
  WheelFrontRightZ/1 -> WheelFrontRight/3

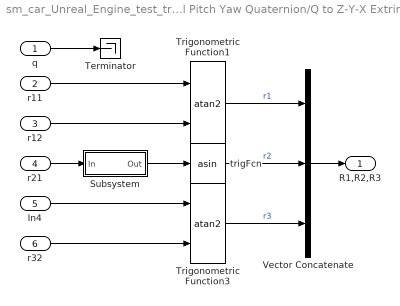
== system sm_car_Unreal_Engine_test_transforms_R19b/Roll Pitch Yaw Quaternion/Q to Z-Y-X Extrinsic/Subsystem ==
  q : Inport
  r11 : Inport  Port=2
  r12 : Inport  Port=3
  r21 : Inport  Port=4
  In4 : Inport  Port=5
  r32 : Inport  Port=6
  Subsystem : Subsystem
  Terminator : Terminator
  Trigonometric Function1 : Trigonometry  Operator=atan2
  Trigonometric Function3 : Trigonometry  Operator=atan2
  Vector Concatenate : Concatenate  NumInputs=3
  trigFcn : Trigonometry  Operator=asin
  R1,R2,R3 : Outport  VectorParamsAs1DForOutWhenUnconnected=off
  wires:
  Vector Concatenate/1 -> R1,R2,R3/1
  r12/1 -> Trigonometric Function1/2
  r21/1 -> Subsystem/1(In)
  r11/1 -> Trigonometric Function1/1
  r32/1 -> Trigonometric Function3/2
  trigFcn/1 -> Vector Concatenate/2  "r2"
  q/1 -> Terminator/1
  Subsystem/1(Out) -> trigFcn/1
  Trigonometric Function3/1 -> Vector Concatenate/3  "r3"
  Trigonometric Function1/1 -> Vector Concatenate/1  "r1"
  In4/1 -> Trigonometric Function3/1

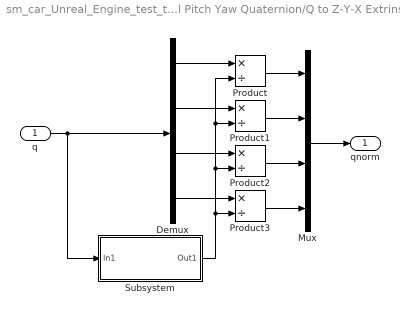
== system sm_car_Unreal_Engine_test_transforms_R19b/Roll Pitch Yaw Quaternion/Q to Z-Y-X Extrinsic/Subsystem1 ==
  q : Inport  Unit=1
  Demux : Demux
  Mux : Mux
  Product{,1..3} (4 alike) : Product  Inputs=*/
  Subsystem : Subsystem
  qnorm : Outport  Unit=1  VectorParamsAs1DForOutWhenUnconnected=off
  wires:
  Product2/1 -> Mux/3
  Demux/2 -> Product1/1
  q/1 -> Subsystem/1(In1), Demux/1
  Demux/4 -> Product3/1
  Demux/3 -> Product2/1
  Product/1 -> Mux/1
  Mux/1 -> qnorm/1
  Subsystem/1(Out1) -> Product3/2, Product2/2, Product/2, Product1/2
  Demux/1 -> Product/1
  Product3/1 -> Mux/4
  Product1/1 -> Mux/2

== system sm_car_Unreal_Engine_test_transforms_R19b/Roll Pitch Yaw Quaternion/Q to Z-Y-X Extrinsic/Subsystem/Subsystem ==
  In : Inport
  If : If  IfExpression=u1 > 1  ElseIfExpressions=u1 < -1
  If Action Subsystem : sharedtransformsys/Protect asincos input/If Action Subsystem  SystemSampleTime=-1  VariantActivationTime=update diagram  Latency=0  AutoFrameSizeCalculation=off
      settings: SourceProductBaseCode=AE,PW,DR,MT,UV,VE
  If Action Subsystem1 : sharedtransformsys/Protect asincos input/If Action Subsystem1  SystemSampleTime=-1  VariantActivationTime=update diagram  Latency=0  AutoFrameSizeCalculation=off
      settings: SourceProductBaseCode=AE,PW,DR,MT,UV,VE
  If Action Subsystem2 : sharedtransformsys/Protect asincos input/If Action Subsystem2  SystemSampleTime=-1  VariantActivationTime=update diagram  Latency=0  AutoFrameSizeCalculation=off
      settings: SourceProductBaseCode=AE,PW,DR,MT,UV,VE
  Merge : Merge  Inputs=3
  Out : Outport  VectorParamsAs1DForOutWhenUnconnected=off
  wires:
  If Action Subsystem1/1 -> Merge/2
  If/1 -> If Action Subsystem/Action
  In/1 -> If/1, If Action Subsystem2/1
  If/3 -> If Action Subsystem2/Action
  If Action Subsystem2/1 -> Merge/3
  If/2 -> If Action Subsystem1/Action
  If Action Subsystem/1 -> Merge/1
  Merge/1 -> Out/1

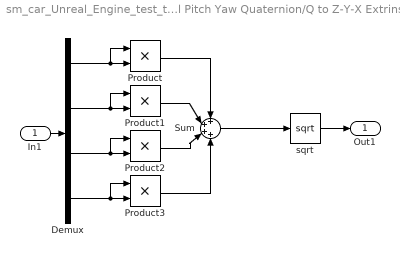
== system sm_car_Unreal_Engine_test_transforms_R19b/Roll Pitch Yaw Quaternion/Q to Z-Y-X Extrinsic/Subsystem1/Subsystem ==
  In1 : Inport
  Demux : Demux
  Product{,1..3} (4 alike) : Product
  Sum : Sum  Inputs=4
  sqrt : Sqrt  AlgorithmType=Newton-Raphson  SaturateOnIntegerOverflow=on
  Out1 : Outport  VectorParamsAs1DForOutWhenUnconnected=off
  wires:
  Sum/1 -> sqrt/1
  sqrt/1 -> Out1/1
  In1/1 -> Demux/1
  Product3/1 -> Sum/4
  Demux/2 -> Product1/1, Product1/2
  Demux/1 -> Product/1, Product/2
  Product2/1 -> Sum/3
  Product/1 -> Sum/1
  Demux/3 -> Product2/1, Product2/2
  Product1/1 -> Sum/2
  Demux/4 -> Product3/1, Product3/2
